simulink model "SensoresDistancia"  (R2023b)
settings: Solver=VariableStepAuto  StartTime=0.0  StopTime=Inf  RelTol=1e-3
libraries: arduinolib x2
settings Model: Creator=Andrés  LastModifiedBy=Andrés

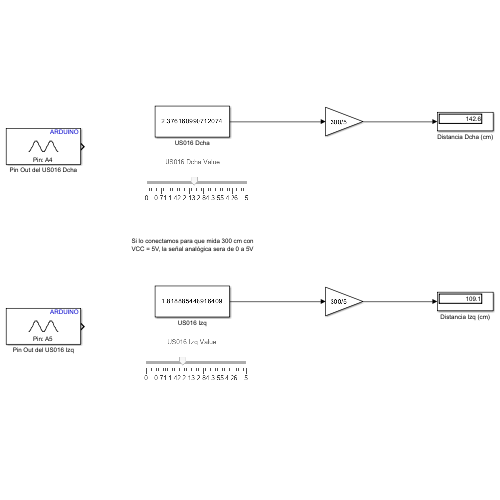
[thumbnail: Simulink's stored preview of the top-level diagram]
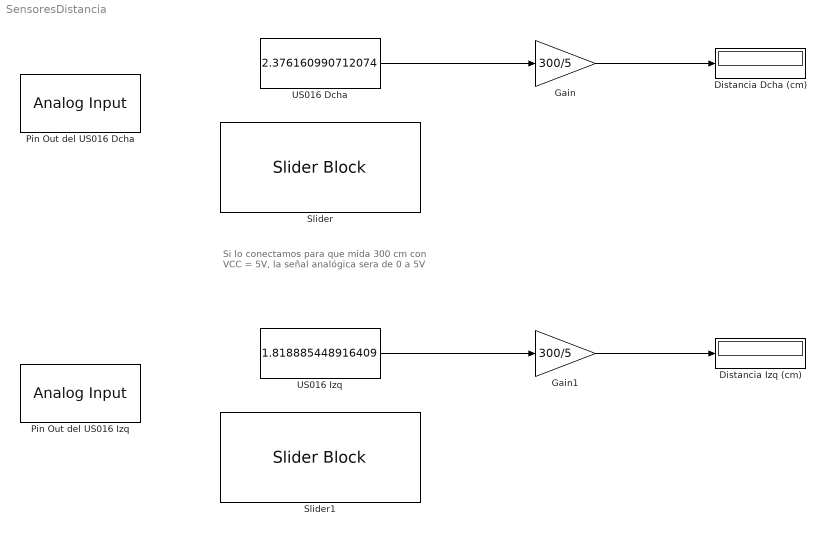
== system SensoresDistancia ==
  note: Si lo conectamos para que mida 300 cm con
      | VCC = 5V, la señal analógica sera de 0 a 5V
  Distancia Dcha (cm) : Display
  Distancia Izq (cm) : Display
  Gain : Gain  Gain=300/5
  Gain1 : Gain  Gain=300/5
  Pin Out del US016 Dcha : arduinolib/Analog Input  pinNumber=4  ReadResultsOnly=off  ConversionTriggerSource=Software  ExternalTriggerType=uint32( 0 )  OutputDataType=uint16  EnableConversionCompleteNotify=off  EnableOuputStatus=off  SampleTime=-1  blockPlatform=arduino
  Pin Out del US016 Izq : arduinolib/Analog Input  pinNumber=5  ReadResultsOnly=off  ConversionTriggerSource=Software  ExternalTriggerType=uint32( 0 )  OutputDataType=uint16  EnableConversionCompleteNotify=off  EnableOuputStatus=off  SampleTime=-1  blockPlatform=arduino
  Slider : SliderBlock  ScaleMax=5
  Slider1 : SliderBlock  ScaleMax=5
  US016 Dcha : Constant  Value=2.376160990712074
  US016 Izq : Constant  Value=1.818885448916409
  wires:
  US016 Dcha/1 -> Gain/1
  Gain/1 -> Distancia Dcha (cm)/1
  US016 Izq/1 -> Gain1/1
  Gain1/1 -> Distancia Izq (cm)/1
